simulink model "flightController"  (R2021a)
settings: Solver=ode3  StartTime=0  StopTime=10  FixedStep=Ts  RelTol=1e-3  EnableMultiTasking=on
undefined symbols (not defined in the file): Controller, ControlvsRed, D_ROLL, delays, DiscIntNeverNeededParam, g, I_ROLL, norm_act, Normalization, P_Pitch, P_ROLL, P_Roll, P_Yaw, P_z, PR_Start, save_time, sts_cnames, time_DisYaw, time_stepsX, time_stepsY, time_stepsZ, Ts, Vehicle, x0, x0_f
libraries: deeplib x5
(part 3 of 4)

== system flightController/Variant Subsystem/ANN/Subsystem2/Subsystem2 ==
  In1 : Inport
  Constant1 : Constant  Value=Ts
  Delay1 : Delay  DelayLength=1  InitialCondition=0
  Divide1 : Product  Inputs=*/
  Sum1 : Sum  Inputs=|+-
  Out1 : Outport
  wires:
  In1/1 -> Delay1/1, Sum1/1
  Constant1/1 -> Divide1/2
  Sum1/1 -> Divide1/1
  Delay1/1 -> Sum1/2
  Divide1/1 -> Out1/1

== system flightController/Variant Subsystem/ANN/Subsystem2/Subsystem3 ==
  In1 : Inport
  Bus Selector2 : BusSelector  OutputSignals=X,Y,Z,yaw,pitch,roll,dx,dy,dz,p,q,r
  Mux : Mux  Inputs=12
  Scope : Scope
  Out5 : Outport
  wires:
  In1/1 -> Bus Selector2/1
  Mux/1 -> Out5/1
  Bus Selector2/1 -> Mux/1  "<X>"
  Bus Selector2/2 -> Mux/2  "<Y>"
  Bus Selector2/3 -> Scope/1, Mux/3  "<Z>"
  Bus Selector2/4 -> Mux/4  "<yaw>"
  Bus Selector2/5 -> Mux/5  "<pitch>"
  Bus Selector2/6 -> Mux/6  "<roll>"
  Bus Selector2/7 -> Mux/7  "<dx>"
  Bus Selector2/8 -> Mux/8  "<dy>"
  Bus Selector2/9 -> Mux/9  "<dz>"
  Bus Selector2/10 -> Mux/10  "<p>"
  Bus Selector2/11 -> Mux/11  "<q>"
  Bus Selector2/12 -> Mux/12  "<r>"

== system flightController/Variant Subsystem/ANN_Feedback/Subsystem1/Subsystem ==
  note: Normalizacion de Sensores
  In1 : Inport
  Bus Selector2 : BusSelector  OutputSignals=ddx,ddy,ddz,p,q,r,altitude_sonar,prs
  Mux : Mux
  Subsystem1 : Subsystem  Commented=on
  Subsystem2 : Subsystem  Commented=on
  Subsystem3 : Subsystem  Commented=on
  Subsystem4 : Subsystem
  Subsystem5 : Subsystem
  Subsystem7 : Subsystem
  Subsystem8 : Subsystem  Commented=on
  Subsystem9 : Subsystem  Commented=on
  Ac_Dz : Outport
  wires:
  In1/1 -> Bus Selector2/1
  Bus Selector2/3 -> Subsystem7/1(<Ac_Dz>)  "<ddz>"
  Bus Selector2/4 -> Subsystem1/1(<Pressure Altitud>)  "<p>"
  Bus Selector2/7 -> Subsystem9/1(<Sonar Altitud>)  "<altitude_sonar>"
  Bus Selector2/8 -> Subsystem3/1(<Pressure Altitud>)  "<prs>"
  Bus Selector2/5 -> Subsystem8/1(<Pressure Altitud>)  "<q>"
  Bus Selector2/6 -> Subsystem2/1(<Pressure Altitud>)  "<r>"
  Mux/1 -> Ac_Dz/1
  Bus Selector2/2 -> Subsystem4/1(<Ac_Dz>)  "<ddy>"
  Bus Selector2/1 -> Subsystem5/1(<Ac_Dz>)  "<ddx>"
  Subsystem2/1(Pressure Altitud) -> Mux/4  "Gyro R"
  Subsystem7/1(Ac_Dz) -> Mux/3  "Ac_Dz"
  Subsystem4/1(Ac_Dz) -> Mux/2  "Ac_Dz"
  Subsystem5/1(Ac_Dz) -> Mux/1  "Ac_Dz"

== system flightController/Variant Subsystem/ANN_Feedback/Subsystem1/Subsystem10 ==
  note: Normalizacion de Sensores
  note: Normalizacion_Z
  note: Normalizacion de ref_Z
  note: Normalizacion_DZ
  note: Normalizacion_Acel_Z
  note: Normalizacion de ref_DZ
  In1 : Inport
  Bus Creator : BusCreator  Inputs=8
  Bus Selector : BusSelector  OutputSignals=Z,Dz,Z_r,Dz_r,Ac_Dz,Sonar Altitud,Pressure Altitud,Acceleracion Z
  Subsystem : Subsystem
  Subsystem2 : Subsystem
  Subsystem3 : Subsystem
  Subsystem4 : Subsystem
  Subsystem6 : Subsystem
  Subsystem7 : Subsystem
  Subsystem8 : Subsystem
  Subsystem9 : Subsystem
  Output : Outport
  wires:
  In1/1 -> Bus Selector/1
  Bus Selector/6 -> Subsystem9/1(<Sonar Altitud>)  "<Sonar Altitud>"
  Subsystem3/1(Z) -> Bus Creator/1
  Subsystem/1(Z_r) -> Bus Creator/3
  Subsystem9/1(Sonar Altitud) -> Bus Creator/6
  Subsystem6/1(Acceleracion Z) -> Bus Creator/8
  Bus Selector/1 -> Subsystem3/1(<Z>)  "<Z>"
  Subsystem7/1(Ac_Dz) -> Bus Creator/5
  Subsystem2/1(Dz_r) -> Bus Creator/4
  Bus Selector/3 -> Subsystem/1(<Z_r>)  "<Z_r>"
  Bus Selector/2 -> Subsystem4/1(<dz>)  "<Dz>"
  Subsystem4/1(Dz) -> Bus Creator/2
  Bus Selector/5 -> Subsystem7/1(<Ac_Dz>)  "<Ac_Dz>"
  Bus Creator/1 -> Output/1
  Subsystem8/1(Pressure Altitud) -> Bus Creator/7
  Bus Selector/4 -> Subsystem2/1(<Dz_r>)  "<Dz_r>"
  Bus Selector/7 -> Subsystem8/1(<Pressure Altitud>)  "<Pressure Altitud>"
  Bus Selector/8 -> Subsystem6/1(<Acel_z>)  "<Acceleracion Z>"

== system flightController/Variant Subsystem/ANN_Feedback/Subsystem1/Subsystem11 ==
  note: Normalizacion de ref_DZ
  note: Normalizacion_Z
  note: Normalizacion de ref_Z
  note: Normalizacion_Acel_Z
  note: Normalizacion de Sensores
  note: Normalizacion_DZ
  In1 : Inport
  Bus Creator : BusCreator  Inputs=8
  Bus Selector1 : BusSelector  OutputSignals=Z,Dz,Z_r,Dz_r,Ac_Dz,Sonar Altitud,Pressure Altitud,Acceleracion Z
  Subsystem : Subsystem
  Subsystem2 : Subsystem
  Subsystem3 : Subsystem
  Subsystem4 : Subsystem
  Subsystem6 : Subsystem
  Subsystem7 : Subsystem
  Subsystem8 : Subsystem
  Subsystem9 : Subsystem
  Output : Outport
  wires:
  Bus Selector1/4 -> Subsystem2/1(<Dz_r>)  "<Dz_r>"
  Bus Selector1/2 -> Subsystem4/1(<dz>)  "<Dz>"
  Bus Selector1/8 -> Subsystem6/1(<Acel_z>)  "<Acceleracion Z>"
  Bus Selector1/1 -> Subsystem3/1(<Z>)  "<Z>"
  In1/1 -> Bus Selector1/1
  Bus Selector1/7 -> Subsystem8/1(<Pressure Altitud>)  "<Pressure Altitud>"
  Subsystem8/1(Pressure Altitud) -> Bus Creator/7
  Subsystem4/1(Dz) -> Bus Creator/2
  Subsystem7/1(Ac_Dz) -> Bus Creator/5
  Bus Selector1/6 -> Subsystem9/1(<Sonar Altitud>)  "<Sonar Altitud>"
  Subsystem9/1(Sonar Altitud) -> Bus Creator/6
  Subsystem2/1(Dz_r) -> Bus Creator/4
  Subsystem6/1(Acceleracion Z) -> Bus Creator/8
  Bus Creator/1 -> Output/1
  Bus Selector1/5 -> Subsystem7/1(<Ac_Dz>)  "<Ac_Dz>"
  Bus Selector1/3 -> Subsystem/1(<Z_r>)  "<Z_r>"
  Subsystem3/1(Z) -> Bus Creator/1
  Subsystem/1(Z_r) -> Bus Creator/3

== system flightController/Variant Subsystem/ANN_Feedback/Subsystem1/Subsystem12 ==
  note: Normalizacion_DZ
  note: Normalizacion de Sensores
  note: Normalizacion_Acel_Z
  note: Normalizacion de ref_Z
  note: Normalizacion_Z
  note: Normalizacion de ref_DZ
  In1 : Inport
  Bus Creator : BusCreator  Inputs=8
  Bus Selector1 : BusSelector  OutputSignals=Z,Dz,Z_r,Dz_r,Ac_Dz,Sonar Altitud,Pressure Altitud,Acceleracion Z
  Subsystem : Subsystem
  Subsystem2 : Subsystem
  Subsystem3 : Subsystem
  Subsystem4 : Subsystem
  Subsystem6 : Subsystem
  Subsystem7 : Subsystem
  Subsystem8 : Subsystem
  Subsystem9 : Subsystem
  Output : Outport
  wires:
  Subsystem/1(Z_r) -> Bus Creator/3
  Subsystem3/1(Z) -> Bus Creator/1
  Bus Selector1/3 -> Subsystem/1(<Z_r>)  "<Z_r>"
  Bus Selector1/5 -> Subsystem7/1(<Ac_Dz>)  "<Ac_Dz>"
  Bus Creator/1 -> Output/1
  Subsystem6/1(Acceleracion Z) -> Bus Creator/8
  Subsystem2/1(Dz_r) -> Bus Creator/4
  Subsystem9/1(Sonar Altitud) -> Bus Creator/6
  Bus Selector1/6 -> Subsystem9/1(<Sonar Altitud>)  "<Sonar Altitud>"
  Subsystem7/1(Ac_Dz) -> Bus Creator/5
  Subsystem4/1(Dz) -> Bus Creator/2
  Subsystem8/1(Pressure Altitud) -> Bus Creator/7
  Bus Selector1/7 -> Subsystem8/1(<Pressure Altitud>)  "<Pressure Altitud>"
  In1/1 -> Bus Selector1/1
  Bus Selector1/1 -> Subsystem3/1(<Z>)  "<Z>"
  Bus Selector1/8 -> Subsystem6/1(<Acel_z>)  "<Acceleracion Z>"
  Bus Selector1/2 -> Subsystem4/1(<dz>)  "<Dz>"
  Bus Selector1/4 -> Subsystem2/1(<Dz_r>)  "<Dz_r>"

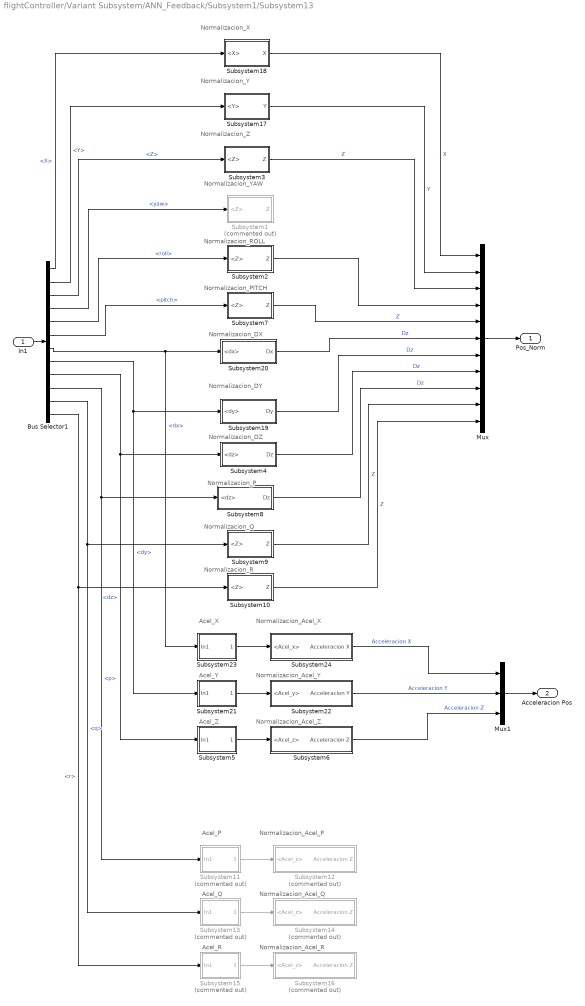
== system flightController/Variant Subsystem/ANN_Feedback/Subsystem1/Subsystem13 ==
  note: Acel_Z
  note: Normalizacion_DZ
  note: Normalizacion_Z
  note: Normalizacion_Acel_Z
  note: Normalizacion_YAW
  note: Normalizacion_ROLL
  note: Normalizacion_PITCH
  note: Normalizacion_P
  note: Normalizacion_Q
  note: Normalizacion_R
  note: Acel_P
  note: Normalizacion_Acel_P
  note: Acel_Q
  note: Normalizacion_Acel_Q
  note: Acel_R
  note: Normalizacion_Acel_R
  note: Normalizacion_Y
  note: Normalizacion_X
  note: Normalizacion_DY
  note: Normalizacion_DX
  note: Acel_Y
  note: Normalizacion_Acel_Y
  note: Acel_X
  note: Normalizacion_Acel_X
  In1 : Inport
  Bus Selector1 : BusSelector  OutputSignals=X,Y,Z,yaw,roll,pitch,dx,dy,dz,p,q,r
  Mux : Mux  Inputs=11
  Mux1 : Mux  Inputs=3
  Subsystem1 : Subsystem  Commented=on
  Subsystem10 : Subsystem
  Subsystem11 : Subsystem  Commented=on
  Subsystem12 : Subsystem  Commented=on
  Subsystem13 : Subsystem  Commented=on
  Subsystem14 : Subsystem  Commented=on
  Subsystem15 : Subsystem  Commented=on
  Subsystem16 : Subsystem  Commented=on
  Subsystem17 : Subsystem
  Subsystem18 : Subsystem
  Subsystem19 : Subsystem
  Subsystem2 : Subsystem
  Subsystem20 : Subsystem
  Subsystem21 : Subsystem
  Subsystem22 : Subsystem
  Subsystem23 : Subsystem
  Subsystem24 : Subsystem
  Subsystem3 : Subsystem
  Subsystem4 : Subsystem
  Subsystem5 : Subsystem
  Subsystem6 : Subsystem
  Subsystem7 : Subsystem
  Subsystem8 : Subsystem
  Subsystem9 : Subsystem
  Pos_Norm : Outport
  Acceleracion Pos : Outport  Port=2
  wires:
  Bus Selector1/3 -> Subsystem3/1(<Z>)  "<Z>"
  Bus Selector1/9 -> Subsystem5/1(In1), Subsystem4/1(<dz>)  "<dz>"
  Subsystem5/1(<Acel_Z>) -> Subsystem6/1(<Acel_z>)
  In1/1 -> Bus Selector1/1
  Bus Selector1/4 -> Subsystem1/1(<Z>)  "<yaw>"
  Bus Selector1/10 -> Subsystem8/1(<dz>), Subsystem11/1(In1)  "<p>"
  Bus Selector1/11 -> Subsystem9/1(<Z>), Subsystem13/1(In1)  "<q>"
  Bus Selector1/12 -> Subsystem10/1(<Z>), Subsystem15/1(In1)  "<r>"
  Mux/1 -> Pos_Norm/1
  Mux1/1 -> Acceleracion Pos/1
  Subsystem11/1(<Acel_Z>) -> Subsystem12/1(<Acel_z>)
  Subsystem13/1(<Acel_Z>) -> Subsystem14/1(<Acel_z>)
  Subsystem15/1(<Acel_Z>) -> Subsystem16/1(<Acel_z>)
  Bus Selector1/5 -> Subsystem2/1(<Z>)  "<roll>"
  Bus Selector1/6 -> Subsystem7/1(<Z>)  "<pitch>"
  Bus Selector1/2 -> Subsystem17/1(<Y>)  "<Y>"
  Bus Selector1/1 -> Subsystem18/1(<X>)  "<X>"
  Bus Selector1/7 -> Subsystem23/1(In1), Subsystem20/1(<dx>)  "<dx>"
  Bus Selector1/8 -> Subsystem21/1(In1), Subsystem19/1(<dy>)  "<dy>"
  Subsystem18/1(X) -> Mux/1  "X"
  Subsystem17/1(Y) -> Mux/2  "Y"
  Subsystem3/1(Z) -> Mux/3  "Z"
  Subsystem2/1(Z) -> Mux/4
  Subsystem7/1(Z) -> Mux/5  "Z"
  Subsystem20/1(Dx) -> Mux/6  "Dz"
  Subsystem19/1(Dy) -> Mux/7  "Dz"
  Subsystem4/1(Dz) -> Mux/8  "Dz"
  Subsystem8/1(Dz) -> Mux/9  "Dz"
  Subsystem9/1(Z) -> Mux/10  "Z"
  Subsystem10/1(Z) -> Mux/11  "Z"
  Subsystem21/1(<Acel_Y>) -> Subsystem22/1(<Acel_y>)
  Subsystem23/1(<Acel_X>) -> Subsystem24/1(<Acel_x>)
  Subsystem22/1(Acceleracion Y) -> Mux1/2  "Acceleracion Y"
  Subsystem24/1(Acceleracion X) -> Mux1/1  "Acceleracion X"
  Subsystem6/1(Acceleracion Z) -> Mux1/3  "Acceleracion Z"

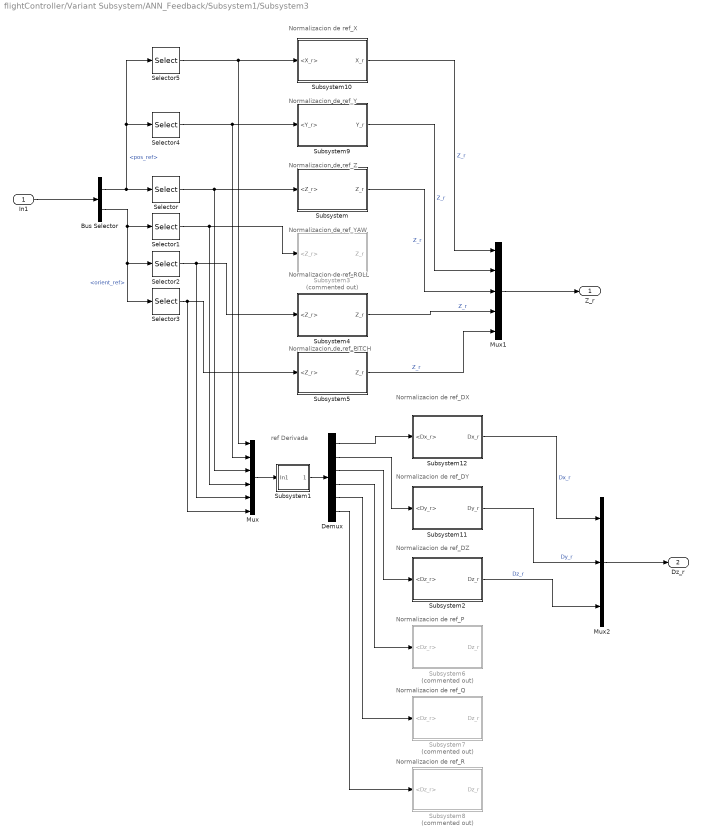
== system flightController/Variant Subsystem/ANN_Feedback/Subsystem1/Subsystem3 ==
  note: Normalizacion de ref_Z
  note: ref
      | Derivada
  note: Normalizacion de ref_DZ
  note: Normalizacion de ref_YAW
  note: Normalizacion de ref_ROLL
  note: Normalizacion de ref_PITCH
  note: Normalizacion de ref_P
  note: Normalizacion de ref_Q
  note: Normalizacion de ref_R
  note: Normalizacion de ref_Y
  note: Normalizacion de ref_X
  note: Normalizacion de ref_DY
  note: Normalizacion de ref_DX
  In1 : Inport
  Bus Selector : BusSelector  OutputSignals=pos_ref,orient_ref
  Demux : Demux  Outputs=6
  Mux : Mux  Inputs=6
  Mux1 : Mux  Inputs=5
  Mux2 : Mux  Inputs=3
  Selector : Selector  InputPortWidth=3  IndexOptions=Index vector (dialog)  Indices=[3]  OutputSizes=1
  Selector1 : Selector  InputPortWidth=3  IndexOptions=Index vector (dialog)  Indices=[1]  OutputSizes=1
  Selector2 : Selector  InputPortWidth=3  IndexOptions=Index vector (dialog)  Indices=[3]  OutputSizes=1
  Selector3 : Selector  InputPortWidth=3  IndexOptions=Index vector (dialog)  Indices=[2]  OutputSizes=1
  Selector4 : Selector  InputPortWidth=3  IndexOptions=Index vector (dialog)  Indices=[2]  OutputSizes=1
  Selector5 : Selector  InputPortWidth=3  IndexOptions=Index vector (dialog)  Indices=[1]  OutputSizes=1
  Subsystem : Subsystem
  Subsystem1 : Subsystem
  Subsystem10 : Subsystem
  Subsystem11 : Subsystem
  Subsystem12 : Subsystem
  Subsystem2 : Subsystem
  Subsystem3 : Subsystem  Commented=on
  Subsystem4 : Subsystem
  Subsystem5 : Subsystem
  Subsystem6 : Subsystem  Commented=on
  Subsystem7 : Subsystem  Commented=on
  Subsystem8 : Subsystem  Commented=on
  Subsystem9 : Subsystem
  Z_r : Outport
  Dz_r : Outport  Port=2
  wires:
  Bus Selector/1 -> Selector5/1, Selector4/1, Selector/1  "<pos_ref>"
  Selector/1 -> Subsystem/1(<Z_r>), Mux/3
  In1/1 -> Bus Selector/1
  Bus Selector/2 -> Selector2/1, Selector3/1, Selector1/1  "<orient_ref>"
  Selector1/1 -> Mux/4, Subsystem3/1(<Z_r>)
  Selector2/1 -> Mux/5, Subsystem4/1(<Z_r>)
  Selector3/1 -> Mux/6, Subsystem5/1(<Z_r>)
  Mux/1 -> Subsystem1/1(In1)
  Subsystem1/1(Out1) -> Demux/1
  Mux1/1 -> Z_r/1
  Mux2/1 -> Dz_r/1
  Selector4/1 -> Mux/2, Subsystem9/1(<Y_r>)
  Selector5/1 -> Mux/1, Subsystem10/1(<X_r>)
  Subsystem10/1(X_r) -> Mux1/1  "Z_r"
  Subsystem9/1(Y_r) -> Mux1/2  "Z_r"
  Subsystem/1(Z_r) -> Mux1/3  "Z_r"
  Subsystem4/1(Z_r) -> Mux1/4  "Z_r"
  Subsystem5/1(Z_r) -> Mux1/5  "Z_r"
  Demux/1 -> Subsystem12/1(<Dx_r>)
  Demux/2 -> Subsystem11/1(<Dy_r>)
  Demux/3 -> Subsystem2/1(<Dz_r>)
  Subsystem12/1(Dx_r) -> Mux2/1  "Dx_r"
  Subsystem11/1(Dy_r) -> Mux2/2  "Dy_r"
  Subsystem2/1(Dz_r) -> Mux2/3  "Dz_r"
  Demux/4 -> Subsystem6/1(<Dz_r>)
  Demux/5 -> Subsystem7/1(<Dz_r>)
  Demux/6 -> Subsystem8/1(<Dz_r>)

== system flightController/Variant Subsystem/ANN_Feedback/Subsystem2/Subsystem ==
  In1 : Inport
  Bus Selector2 : BusSelector  OutputSignals=ddx,ddy,ddz,p,q,r,altitude_sonar,prs,vbat_V,vbat_percentage
  Cast To Single : DataTypeConversion  OutDataTypeStr=single
  Mux : Mux  Inputs=10
  Scope : Scope
  Out5 : Outport
  wires:
  In1/1 -> Bus Selector2/1
  Bus Selector2/1 -> Mux/1  "<ddx>"
  Bus Selector2/2 -> Mux/2  "<ddy>"
  Bus Selector2/3 -> Mux/3  "<ddz>"
  Bus Selector2/4 -> Mux/4  "<p>"
  Bus Selector2/5 -> Mux/5  "<q>"
  Bus Selector2/6 -> Mux/6  "<r>"
  Bus Selector2/7 -> Mux/7  "<altitude_sonar>"
  Bus Selector2/8 -> Mux/8  "<prs>"
  Bus Selector2/9 -> Mux/9  "<vbat_V>"
  Mux/1 -> Scope/1, Out5/1
  Bus Selector2/10 -> Cast To Single/1  "<vbat_percentage>"
  Cast To Single/1 -> Mux/10

== system flightController/Variant Subsystem/ANN_Feedback/Subsystem2/Subsystem1 ==
  In1 : Inport
  Constant1 : Constant  Value=Ts
  Delay1 : Delay  DelayLength=1  InitialCondition=0
  Divide1 : Product  Inputs=*/
  Sum1 : Sum  Inputs=|+-
  Out1 : Outport
  wires:
  In1/1 -> Delay1/1, Sum1/1
  Constant1/1 -> Divide1/2
  Sum1/1 -> Divide1/1
  Delay1/1 -> Sum1/2
  Divide1/1 -> Out1/1

== system flightController/Variant Subsystem/ANN_Feedback/Subsystem2/Subsystem2 ==
  In1 : Inport
  Constant1 : Constant  Value=Ts
  Delay1 : Delay  DelayLength=1  InitialCondition=0
  Divide1 : Product  Inputs=*/
  Sum1 : Sum  Inputs=|+-
  Out1 : Outport
  wires:
  In1/1 -> Delay1/1, Sum1/1
  Constant1/1 -> Divide1/2
  Sum1/1 -> Divide1/1
  Delay1/1 -> Sum1/2
  Divide1/1 -> Out1/1

== system flightController/Variant Subsystem/ANN_Feedback/Subsystem2/Subsystem3 ==
  In1 : Inport
  Bus Selector2 : BusSelector  OutputSignals=X,Y,Z,yaw,pitch,roll,dx,dy,dz,p,q,r
  Mux : Mux  Inputs=12
  Scope : Scope
  Out5 : Outport
  wires:
  In1/1 -> Bus Selector2/1
  Mux/1 -> Out5/1
  Bus Selector2/1 -> Mux/1  "<X>"
  Bus Selector2/2 -> Mux/2  "<Y>"
  Bus Selector2/3 -> Scope/1, Mux/3  "<Z>"
  Bus Selector2/4 -> Mux/4  "<yaw>"
  Bus Selector2/5 -> Mux/5  "<pitch>"
  Bus Selector2/6 -> Mux/6  "<roll>"
  Bus Selector2/7 -> Mux/7  "<dx>"
  Bus Selector2/8 -> Mux/8  "<dy>"
  Bus Selector2/9 -> Mux/9  "<dz>"
  Bus Selector2/10 -> Mux/10  "<p>"
  Bus Selector2/11 -> Mux/11  "<q>"
  Bus Selector2/12 -> Mux/12  "<r>"

== system flightController/Variant Subsystem/LSTM/Subsystem2/Subsystem ==
  In1 : Inport
  Bus Selector2 : BusSelector  OutputSignals=ddx,ddy,ddz,p,q,r,altitude_sonar,prs,vbat_V,vbat_percentage
  Cast To Single : DataTypeConversion  OutDataTypeStr=single
  Mux : Mux  Inputs=10
  Scope : Scope
  Out5 : Outport
  wires:
  In1/1 -> Bus Selector2/1
  Bus Selector2/1 -> Mux/1  "<ddx>"
  Bus Selector2/2 -> Mux/2  "<ddy>"
  Bus Selector2/3 -> Mux/3  "<ddz>"
  Bus Selector2/4 -> Mux/4  "<p>"
  Bus Selector2/5 -> Mux/5  "<q>"
  Bus Selector2/6 -> Mux/6  "<r>"
  Bus Selector2/7 -> Mux/7  "<altitude_sonar>"
  Bus Selector2/8 -> Mux/8  "<prs>"
  Bus Selector2/9 -> Mux/9  "<vbat_V>"
  Mux/1 -> Scope/1, Out5/1
  Bus Selector2/10 -> Cast To Single/1  "<vbat_percentage>"
  Cast To Single/1 -> Mux/10

== system flightController/Variant Subsystem/LSTM/Subsystem2/Subsystem1 ==
  In1 : Inport
  Constant1 : Constant  Value=Ts
  Delay1 : Delay  DelayLength=1  InitialCondition=0
  Divide1 : Product  Inputs=*/
  Sum1 : Sum  Inputs=|+-
  Out1 : Outport
  wires:
  In1/1 -> Delay1/1, Sum1/1
  Constant1/1 -> Divide1/2
  Sum1/1 -> Divide1/1
  Delay1/1 -> Sum1/2
  Divide1/1 -> Out1/1

== system flightController/Variant Subsystem/LSTM/Subsystem2/Subsystem2 ==
  In1 : Inport
  Constant1 : Constant  Value=Ts
  Delay1 : Delay  DelayLength=1  InitialCondition=0
  Divide1 : Product  Inputs=*/
  Sum1 : Sum  Inputs=|+-
  Out1 : Outport
  wires:
  In1/1 -> Delay1/1, Sum1/1
  Constant1/1 -> Divide1/2
  Sum1/1 -> Divide1/1
  Delay1/1 -> Sum1/2
  Divide1/1 -> Out1/1

== system flightController/Variant Subsystem/LSTM/Subsystem2/Subsystem3 ==
  In1 : Inport
  Bus Selector2 : BusSelector  OutputSignals=X,Y,Z,yaw,pitch,roll,dx,dy,dz,p,q,r
  Mux : Mux  Inputs=12
  Scope : Scope
  Out5 : Outport
  wires:
  In1/1 -> Bus Selector2/1
  Mux/1 -> Out5/1
  Bus Selector2/1 -> Mux/1  "<X>"
  Bus Selector2/2 -> Mux/2  "<Y>"
  Bus Selector2/3 -> Scope/1, Mux/3  "<Z>"
  Bus Selector2/4 -> Mux/4  "<yaw>"
  Bus Selector2/7 -> Mux/7  "<dx>"
  Bus Selector2/8 -> Mux/8  "<dy>"
  Bus Selector2/9 -> Mux/9  "<dz>"
  Bus Selector2/10 -> Mux/10  "<p>"
  Bus Selector2/11 -> Mux/11  "<q>"
  Bus Selector2/12 -> Mux/12  "<r>"
  Bus Selector2/6 -> Mux/5  "<roll>"
  Bus Selector2/5 -> Mux/6  "<pitch>"

== system flightController/Variant Subsystem/LSTM/Subsystem3/Subsystem ==
  In1 : Inport
  Bus Selector2 : BusSelector  OutputSignals=ddx,ddy,ddz,p,q,r,altitude_sonar,prs,vbat_V,vbat_percentage
  Cast To Single : DataTypeConversion  OutDataTypeStr=single
  Mux : Mux  Inputs=10
  Out5 : Outport
  wires:
  In1/1 -> Bus Selector2/1
  Bus Selector2/1 -> Mux/1  "<ddx>"
  Bus Selector2/2 -> Mux/2  "<ddy>"
  Bus Selector2/3 -> Mux/3  "<ddz>"
  Bus Selector2/4 -> Mux/4  "<p>"
  Bus Selector2/5 -> Mux/5  "<q>"
  Bus Selector2/6 -> Mux/6  "<r>"
  Bus Selector2/7 -> Mux/7  "<altitude_sonar>"
  Bus Selector2/8 -> Mux/8  "<prs>"
  Bus Selector2/9 -> Mux/9  "<vbat_V>"
  Mux/1 -> Out5/1
  Bus Selector2/10 -> Cast To Single/1  "<vbat_percentage>"
  Cast To Single/1 -> Mux/10

== system flightController/Variant Subsystem/LSTM/Subsystem3/Subsystem1 ==
  In1 : Inport
  Constant1 : Constant  Value=Ts
  Delay1 : Delay  DelayLength=1  InitialCondition=0
  Divide1 : Product  Inputs=*/
  Sum1 : Sum  Inputs=|+-
  Out1 : Outport
  wires:
  In1/1 -> Delay1/1, Sum1/1
  Constant1/1 -> Divide1/2
  Sum1/1 -> Divide1/1
  Delay1/1 -> Sum1/2
  Divide1/1 -> Out1/1

== system flightController/Variant Subsystem/LSTM/Subsystem3/Subsystem2 ==
  In1 : Inport
  Constant1 : Constant  Value=Ts
  Delay1 : Delay  DelayLength=1  InitialCondition=0
  Divide1 : Product  Inputs=*/
  Sum1 : Sum  Inputs=|+-
  Out1 : Outport
  wires:
  In1/1 -> Delay1/1, Sum1/1
  Constant1/1 -> Divide1/2
  Sum1/1 -> Divide1/1
  Delay1/1 -> Sum1/2
  Divide1/1 -> Out1/1

== system flightController/Variant Subsystem/LSTM/Subsystem3/Subsystem3 ==
  In1 : Inport
  Bus Selector2 : BusSelector  OutputSignals=X,Y,Z,yaw,pitch,roll,dx,dy,dz,p,q,r
  Mux : Mux  Inputs=12
  Scope : Scope
  Out5 : Outport
  wires:
  In1/1 -> Bus Selector2/1
  Mux/1 -> Out5/1
  Bus Selector2/1 -> Mux/1  "<X>"
  Bus Selector2/2 -> Mux/2  "<Y>"
  Bus Selector2/3 -> Scope/1, Mux/3  "<Z>"
  Bus Selector2/4 -> Mux/4  "<yaw>"
  Bus Selector2/5 -> Mux/5  "<pitch>"
  Bus Selector2/6 -> Mux/6  "<roll>"
  Bus Selector2/7 -> Mux/7  "<dx>"
  Bus Selector2/8 -> Mux/8  "<dy>"
  Bus Selector2/9 -> Mux/9  "<dz>"
  Bus Selector2/10 -> Mux/10  "<p>"
  Bus Selector2/11 -> Mux/11  "<q>"
  Bus Selector2/12 -> Mux/12  "<r>"

== system flightController/Variant Subsystem/ANN/Subsystem/Subsystem/Subsystem1 ==
  <Pressure Altitud> : Inport
  Constant : Constant  Value=Normalization(13,2)
  Gain : Gain  Gain=1/(Normalization(13,1)-Normalization(13,2))
  Sum : Sum  Inputs=|+-
  Pressure Altitud : Outport
  wires:
  <Pressure Altitud>/1 -> Sum/1
  Sum/1 -> Gain/1
  Constant/1 -> Sum/2
  Gain/1 -> Pressure Altitud/1

== system flightController/Variant Subsystem/ANN/Subsystem/Subsystem/Subsystem2 ==
  <Pressure Altitud> : Inport
  Constant : Constant  Value=Normalization(15,2)
  Gain : Gain  Gain=1/(Normalization(15,1)-Normalization(15,2))
  Sum : Sum  Inputs=|+-
  Pressure Altitud : Outport
  wires:
  <Pressure Altitud>/1 -> Sum/1
  Sum/1 -> Gain/1
  Constant/1 -> Sum/2
  Gain/1 -> Pressure Altitud/1

== system flightController/Variant Subsystem/ANN/Subsystem/Subsystem/Subsystem3 ==
  <Pressure Altitud> : Inport
  Constant : Constant  Value=Normalization(17,2)
  Gain : Gain  Gain=1/(Normalization(17,1)-Normalization(17,2))
  Sum : Sum  Inputs=|+-
  Pressure Altitud : Outport
  wires:
  <Pressure Altitud>/1 -> Sum/1
  Sum/1 -> Gain/1
  Constant/1 -> Sum/2
  Gain/1 -> Pressure Altitud/1

== system flightController/Variant Subsystem/ANN/Subsystem/Subsystem/Subsystem7 ==
  <Ac_Dz> : Inport
  Constant : Constant  Value=Normalization(12,2)
  Gain : Gain  Gain=1/(Normalization(12,1)-Normalization(12,2))
  Sum : Sum  Inputs=|+-
  Ac_Dz : Outport
  wires:
  <Ac_Dz>/1 -> Sum/1
  Sum/1 -> Gain/1
  Constant/1 -> Sum/2
  Gain/1 -> Ac_Dz/1

== system flightController/Variant Subsystem/ANN/Subsystem/Subsystem/Subsystem8 ==
  <Pressure Altitud> : Inport
  Constant : Constant  Value=Normalization(14,2)
  Gain : Gain  Gain=1/(Normalization(14,1)-Normalization(14,2))
  Sum : Sum  Inputs=|+-
  Pressure Altitud : Outport
  wires:
  <Pressure Altitud>/1 -> Sum/1
  Sum/1 -> Gain/1
  Constant/1 -> Sum/2
  Gain/1 -> Pressure Altitud/1

== system flightController/Variant Subsystem/ANN/Subsystem/Subsystem/Subsystem9 ==
  <Sonar Altitud> : Inport
  Constant : Constant  Value=Normalization(16,2)
  Gain : Gain  Gain=1/(Normalization(16,1)-Normalization(16,2))
  Scope : Scope
  Sum : Sum  Inputs=|+-
  Sonar Altitud : Outport
  wires:
  <Sonar Altitud>/1 -> Scope/1, Sum/1
  Sum/1 -> Gain/1
  Constant/1 -> Sum/2
  Gain/1 -> Sonar Altitud/1

== system flightController/Variant Subsystem/ANN/Subsystem/Subsystem10/Subsystem ==
  <Z_r> : Inport
  Constant : Constant  Value=Normalization(10,2)
  Gain : Gain  Gain=1/(Normalization(10,1)-Normalization(10,2))
  Sum : Sum  Inputs=|+-
  Z_r : Outport
  wires:
  <Z_r>/1 -> Sum/1
  Sum/1 -> Gain/1
  Constant/1 -> Sum/2
  Gain/1 -> Z_r/1

== system flightController/Variant Subsystem/ANN/Subsystem/Subsystem10/Subsystem2 ==
  <Dz_r> : Inport
  Constant : Constant  Value=Normalization(14,2)
  Gain : Gain  Gain=1/(Normalization(14,1)-Normalization(14,2))
  Sum : Sum  Inputs=|+-
  Dz_r : Outport
  wires:
  <Dz_r>/1 -> Sum/1
  Sum/1 -> Gain/1
  Constant/1 -> Sum/2
  Gain/1 -> Dz_r/1

== system flightController/Variant Subsystem/ANN/Subsystem/Subsystem10/Subsystem3 ==
  <Z> : Inport
  Constant : Constant  Value=Normalization(2,2)
  Gain : Gain  Gain=1/(Normalization(2,1)-Normalization(2,2))
  Sum : Sum  Inputs=|+-
  Z : Outport
  wires:
  Constant/1 -> Sum/2
  Sum/1 -> Gain/1
  Gain/1 -> Z/1
  <Z>/1 -> Sum/1

== system flightController/Variant Subsystem/ANN/Subsystem/Subsystem10/Subsystem4 ==
  <dz> : Inport
  Constant : Constant  Value=Normalization(5,2)
  Gain : Gain  Gain=1/(Normalization(5,1)-Normalization(5,2))
  Sum : Sum  Inputs=|+-
  Dz : Outport
  wires:
  Gain/1 -> Dz/1
  Constant/1 -> Sum/2
  <dz>/1 -> Sum/1
  Sum/1 -> Gain/1

== system flightController/Variant Subsystem/ANN/Subsystem/Subsystem10/Subsystem6 ==
  <Acel_z> : Inport
  Constant : Constant  Value=Normalization(30,2)
  Gain : Gain  Gain=1/(Normalization(30,1)-Normalization(30,2))
  Sum : Sum  Inputs=|+-
  Acceleracion Z : Outport
  wires:
  Gain/1 -> Acceleracion Z/1
  Constant/1 -> Sum/2
  <Acel_z>/1 -> Sum/1
  Sum/1 -> Gain/1

== system flightController/Variant Subsystem/ANN/Subsystem/Subsystem10/Subsystem7 ==
  <Ac_Dz> : Inport
  Constant : Constant  Value=Normalization(18,2)
  Gain : Gain  Gain=1/(Normalization(18,1)-Normalization(18,2))
  Sum : Sum  Inputs=|+-
  Ac_Dz : Outport
  wires:
  <Ac_Dz>/1 -> Sum/1
  Sum/1 -> Gain/1
  Constant/1 -> Sum/2
  Gain/1 -> Ac_Dz/1

== system flightController/Variant Subsystem/ANN/Subsystem/Subsystem10/Subsystem8 ==
  <Pressure Altitud> : Inport
  Constant : Constant  Value=Normalization(26,2)
  Gain : Gain  Gain=1/(Normalization(26,1)-Normalization(26,2))
  Sum : Sum  Inputs=|+-
  Pressure Altitud : Outport
  wires:
  <Pressure Altitud>/1 -> Sum/1
  Sum/1 -> Gain/1
  Constant/1 -> Sum/2
  Gain/1 -> Pressure Altitud/1

== system flightController/Variant Subsystem/ANN/Subsystem/Subsystem10/Subsystem9 ==
  <Sonar Altitud> : Inport
  Constant : Constant  Value=Normalization(22,2)
  Gain : Gain  Gain=1/(Normalization(22,1)-Normalization(22,2))
  Sum : Sum  Inputs=|+-
  Sonar Altitud : Outport
  wires:
  <Sonar Altitud>/1 -> Sum/1
  Sum/1 -> Gain/1
  Constant/1 -> Sum/2
  Gain/1 -> Sonar Altitud/1

== system flightController/Variant Subsystem/ANN/Subsystem/Subsystem11/Subsystem ==
  <Z_r> : Inport
  Constant : Constant  Value=Normalization(10,2)
  Gain : Gain  Gain=1/(Normalization(10,1)-Normalization(10,2))
  Sum : Sum  Inputs=|+-
  Z_r : Outport
  wires:
  <Z_r>/1 -> Sum/1
  Sum/1 -> Gain/1
  Constant/1 -> Sum/2
  Gain/1 -> Z_r/1

== system flightController/Variant Subsystem/ANN/Subsystem/Subsystem11/Subsystem2 ==
  <Dz_r> : Inport
  Constant : Constant  Value=Normalization(14,2)
  Gain : Gain  Gain=1/(Normalization(14,1)-Normalization(14,2))
  Sum : Sum  Inputs=|+-
  Dz_r : Outport
  wires:
  <Dz_r>/1 -> Sum/1
  Sum/1 -> Gain/1
  Constant/1 -> Sum/2
  Gain/1 -> Dz_r/1

== system flightController/Variant Subsystem/ANN/Subsystem/Subsystem11/Subsystem3 ==
  <Z> : Inport
  Constant : Constant  Value=Normalization(3,2)
  Gain : Gain  Gain=1/(Normalization(3,1)-Normalization(3,2))
  Sum : Sum  Inputs=|+-
  Z : Outport
  wires:
  Constant/1 -> Sum/2
  Sum/1 -> Gain/1
  Gain/1 -> Z/1
  <Z>/1 -> Sum/1

== system flightController/Variant Subsystem/ANN/Subsystem/Subsystem11/Subsystem4 ==
  <dz> : Inport
  Constant : Constant  Value=Normalization(6,2)
  Gain : Gain  Gain=1/(Normalization(6,1)-Normalization(6,2))
  Sum : Sum  Inputs=|+-
  Dz : Outport
  wires:
  Gain/1 -> Dz/1
  Constant/1 -> Sum/2
  <dz>/1 -> Sum/1
  Sum/1 -> Gain/1

== system flightController/Variant Subsystem/ANN/Subsystem/Subsystem11/Subsystem6 ==
  <Acel_z> : Inport
  Constant : Constant  Value=Normalization(30,2)
  Gain : Gain  Gain=1/(Normalization(30,1)-Normalization(30,2))
  Sum : Sum  Inputs=|+-
  Acceleracion Z : Outport
  wires:
  Gain/1 -> Acceleracion Z/1
  Constant/1 -> Sum/2
  <Acel_z>/1 -> Sum/1
  Sum/1 -> Gain/1

== system flightController/Variant Subsystem/ANN/Subsystem/Subsystem11/Subsystem7 ==
  <Ac_Dz> : Inport
  Constant : Constant  Value=Normalization(18,2)
  Gain : Gain  Gain=1/(Normalization(18,1)-Normalization(18,2))
  Sum : Sum  Inputs=|+-
  Ac_Dz : Outport
  wires:
  <Ac_Dz>/1 -> Sum/1
  Sum/1 -> Gain/1
  Constant/1 -> Sum/2
  Gain/1 -> Ac_Dz/1

== system flightController/Variant Subsystem/ANN/Subsystem/Subsystem11/Subsystem8 ==
  <Pressure Altitud> : Inport
  Constant : Constant  Value=Normalization(26,2)
  Gain : Gain  Gain=1/(Normalization(26,1)-Normalization(26,2))
  Sum : Sum  Inputs=|+-
  Pressure Altitud : Outport
  wires:
  <Pressure Altitud>/1 -> Sum/1
  Sum/1 -> Gain/1
  Constant/1 -> Sum/2
  Gain/1 -> Pressure Altitud/1

== system flightController/Variant Subsystem/ANN/Subsystem/Subsystem11/Subsystem9 ==
  <Sonar Altitud> : Inport
  Constant : Constant  Value=Normalization(22,2)
  Gain : Gain  Gain=1/(Normalization(22,1)-Normalization(22,2))
  Sum : Sum  Inputs=|+-
  Sonar Altitud : Outport
  wires:
  <Sonar Altitud>/1 -> Sum/1
  Sum/1 -> Gain/1
  Constant/1 -> Sum/2
  Gain/1 -> Sonar Altitud/1

== system flightController/Variant Subsystem/ANN/Subsystem/Subsystem12/Subsystem ==
  <Z_r> : Inport
  Constant : Constant  Value=Normalization(10,2)
  Gain : Gain  Gain=1/(Normalization(10,1)-Normalization(10,2))
  Sum : Sum  Inputs=|+-
  Z_r : Outport
  wires:
  Gain/1 -> Z_r/1
  Constant/1 -> Sum/2
  Sum/1 -> Gain/1
  <Z_r>/1 -> Sum/1

== system flightController/Variant Subsystem/ANN/Subsystem/Subsystem12/Subsystem2 ==
  <Dz_r> : Inport
  Constant : Constant  Value=Normalization(14,2)
  Gain : Gain  Gain=1/(Normalization(14,1)-Normalization(14,2))
  Sum : Sum  Inputs=|+-
  Dz_r : Outport
  wires:
  Gain/1 -> Dz_r/1
  Constant/1 -> Sum/2
  Sum/1 -> Gain/1
  <Dz_r>/1 -> Sum/1

== system flightController/Variant Subsystem/ANN/Subsystem/Subsystem12/Subsystem3 ==
  <Z> : Inport
  Constant : Constant  Value=Normalization(3,2)
  Gain : Gain  Gain=1/(Normalization(3,1)-Normalization(3,2))
  Sum : Sum  Inputs=|+-
  Z : Outport
  wires:
  <Z>/1 -> Sum/1
  Gain/1 -> Z/1
  Sum/1 -> Gain/1
  Constant/1 -> Sum/2

== system flightController/Variant Subsystem/ANN/Subsystem/Subsystem12/Subsystem4 ==
  <dz> : Inport
  Constant : Constant  Value=Normalization(6,2)
  Gain : Gain  Gain=1/(Normalization(6,1)-Normalization(6,2))
  Sum : Sum  Inputs=|+-
  Dz : Outport
  wires:
  Sum/1 -> Gain/1
  <dz>/1 -> Sum/1
  Constant/1 -> Sum/2
  Gain/1 -> Dz/1

== system flightController/Variant Subsystem/ANN/Subsystem/Subsystem12/Subsystem6 ==
  <Acel_z> : Inport
  Constant : Constant  Value=Normalization(30,2)
  Gain : Gain  Gain=1/(Normalization(30,1)-Normalization(30,2))
  Sum : Sum  Inputs=|+-
  Acceleracion Z : Outport
  wires:
  Sum/1 -> Gain/1
  <Acel_z>/1 -> Sum/1
  Constant/1 -> Sum/2
  Gain/1 -> Acceleracion Z/1

== system flightController/Variant Subsystem/ANN/Subsystem/Subsystem12/Subsystem7 ==
  <Ac_Dz> : Inport
  Constant : Constant  Value=Normalization(18,2)
  Gain : Gain  Gain=1/(Normalization(18,1)-Normalization(18,2))
  Sum : Sum  Inputs=|+-
  Ac_Dz : Outport
  wires:
  Gain/1 -> Ac_Dz/1
  Constant/1 -> Sum/2
  Sum/1 -> Gain/1
  <Ac_Dz>/1 -> Sum/1

== system flightController/Variant Subsystem/ANN/Subsystem/Subsystem12/Subsystem8 ==
  <Pressure Altitud> : Inport
  Constant : Constant  Value=Normalization(26,2)
  Gain : Gain  Gain=1/(Normalization(26,1)-Normalization(26,2))
  Sum : Sum  Inputs=|+-
  Pressure Altitud : Outport
  wires:
  Gain/1 -> Pressure Altitud/1
  Constant/1 -> Sum/2
  Sum/1 -> Gain/1
  <Pressure Altitud>/1 -> Sum/1

== system flightController/Variant Subsystem/ANN/Subsystem/Subsystem12/Subsystem9 ==
  <Sonar Altitud> : Inport
  Constant : Constant  Value=Normalization(22,2)
  Gain : Gain  Gain=1/(Normalization(22,1)-Normalization(22,2))
  Sum : Sum  Inputs=|+-
  Sonar Altitud : Outport
  wires:
  Gain/1 -> Sonar Altitud/1
  Constant/1 -> Sum/2
  Sum/1 -> Gain/1
  <Sonar Altitud>/1 -> Sum/1

== system flightController/Variant Subsystem/ANN/Subsystem/Subsystem13/Subsystem1 ==
  <Z> : Inport
  Constant : Constant  Value=Normalization(2,2)
  Gain : Gain  Gain=1/(Normalization(2,1)-Normalization(2,2))
  Sum : Sum  Inputs=|+-
  Z : Outport
  wires:
  Constant/1 -> Sum/2
  Sum/1 -> Gain/1
  Gain/1 -> Z/1
  <Z>/1 -> Sum/1

== system flightController/Variant Subsystem/ANN/Subsystem/Subsystem13/Subsystem10 ==
  <Z> : Inport
  Constant : Constant  Value=Normalization(7,2)
  Gain : Gain  Gain=1/(Normalization(7,1)-Normalization(7,2))
  Sum : Sum  Inputs=|+-
  Z : Outport
  wires:
  Constant/1 -> Sum/2
  Sum/1 -> Gain/1
  Gain/1 -> Z/1
  <Z>/1 -> Sum/1

== system flightController/Variant Subsystem/ANN/Subsystem/Subsystem13/Subsystem11 ==
  In1 : Inport
  Constant1 : Constant  Value=Ts
  Delay1 : Delay  DelayLength=1  InitialCondition=0
  Divide1 : Product  Inputs=*/
  Sum1 : Sum  Inputs=|+-
  <Acel_Z> : Outport
  wires:
  Divide1/1 -> <Acel_Z>/1
  Delay1/1 -> Sum1/2
  Sum1/1 -> Divide1/1
  Constant1/1 -> Divide1/2
  In1/1 -> Sum1/1, Delay1/1

== system flightController/Variant Subsystem/ANN/Subsystem/Subsystem13/Subsystem12 ==
  <Acel_z> : Inport
  Constant : Constant  Value=Normalization(24,2)
  Gain : Gain  Gain=1/(Normalization(24,1)-Normalization(24,2))
  Sum : Sum  Inputs=|+-
  Acceleracion Z : Outport
  wires:
  Sum/1 -> Gain/1
  <Acel_z>/1 -> Sum/1
  Constant/1 -> Sum/2
  Gain/1 -> Acceleracion Z/1

== system flightController/Variant Subsystem/ANN/Subsystem/Subsystem13/Subsystem13 ==
  In1 : Inport
  Constant1 : Constant  Value=Ts
  Delay1 : Delay  DelayLength=1  InitialCondition=0
  Divide1 : Product  Inputs=*/
  Sum1 : Sum  Inputs=|+-
  <Acel_Z> : Outport
  wires:
  Divide1/1 -> <Acel_Z>/1
  Delay1/1 -> Sum1/2
  Sum1/1 -> Divide1/1
  Constant1/1 -> Divide1/2
  In1/1 -> Sum1/1, Delay1/1

== system flightController/Variant Subsystem/ANN/Subsystem/Subsystem13/Subsystem14 ==
  <Acel_z> : Inport
  Constant : Constant  Value=Normalization(25,2)
  Gain : Gain  Gain=1/(Normalization(25,1)-Normalization(25,2))
  Sum : Sum  Inputs=|+-
  Acceleracion Z : Outport
  wires:
  Sum/1 -> Gain/1
  <Acel_z>/1 -> Sum/1
  Constant/1 -> Sum/2
  Gain/1 -> Acceleracion Z/1

== system flightController/Variant Subsystem/ANN/Subsystem/Subsystem13/Subsystem15 ==
  In1 : Inport
  Constant1 : Constant  Value=Ts
  Delay1 : Delay  DelayLength=1  InitialCondition=0
  Divide1 : Product  Inputs=*/
  Sum1 : Sum  Inputs=|+-
  <Acel_Z> : Outport
  wires:
  Divide1/1 -> <Acel_Z>/1
  Delay1/1 -> Sum1/2
  Sum1/1 -> Divide1/1
  Constant1/1 -> Divide1/2
  In1/1 -> Sum1/1, Delay1/1

== system flightController/Variant Subsystem/ANN/Subsystem/Subsystem13/Subsystem16 ==
  <Acel_z> : Inport
  Constant : Constant  Value=Normalization(26,2)
  Gain : Gain  Gain=1/(Normalization(26,1)-Normalization(26,2))
  Sum : Sum  Inputs=|+-
  Acceleracion Z : Outport
  wires:
  Sum/1 -> Gain/1
  <Acel_z>/1 -> Sum/1
  Constant/1 -> Sum/2
  Gain/1 -> Acceleracion Z/1

== system flightController/Variant Subsystem/ANN/Subsystem/Subsystem13/Subsystem2 ==
  <Z> : Inport
  Constant : Constant  Value=Normalization(2,2)
  Gain : Gain  Gain=1/(Normalization(2,1)-Normalization(2,2))
  Sum : Sum  Inputs=|+-
  Z : Outport
  wires:
  Constant/1 -> Sum/2
  Sum/1 -> Gain/1
  Gain/1 -> Z/1
  <Z>/1 -> Sum/1

== system flightController/Variant Subsystem/ANN/Subsystem/Subsystem13/Subsystem3 ==
  <Z> : Inport
  Constant : Constant  Value=Normalization(1,2)
  Gain : Gain  Gain=1/(Normalization(1,1)-Normalization(1,2))
  Sum : Sum  Inputs=|+-
  Z : Outport
  wires:
  Constant/1 -> Sum/2
  Sum/1 -> Gain/1
  Gain/1 -> Z/1
  <Z>/1 -> Sum/1

== system flightController/Variant Subsystem/ANN/Subsystem/Subsystem13/Subsystem4 ==
  <dz> : Inport
  Constant : Constant  Value=Normalization(4,2)
  Gain : Gain  Gain=1/(Normalization(4,1)-Normalization(4,2))
  Sum : Sum  Inputs=|+-
  Dz : Outport
  wires:
  Gain/1 -> Dz/1
  Constant/1 -> Sum/2
  <dz>/1 -> Sum/1
  Sum/1 -> Gain/1

== system flightController/Variant Subsystem/ANN/Subsystem/Subsystem13/Subsystem5 ==
  In1 : Inport
  Constant1 : Constant  Value=Ts
  Delay1 : Delay  DelayLength=1  InitialCondition=0
  Divide1 : Product  Inputs=*/
  Sum1 : Sum  Inputs=|+-
  <Acel_Z> : Outport
  wires:
  In1/1 -> Delay1/1, Sum1/1
  Constant1/1 -> Divide1/2
  Sum1/1 -> Divide1/1
  Delay1/1 -> Sum1/2
  Divide1/1 -> <Acel_Z>/1

== system flightController/Variant Subsystem/ANN/Subsystem/Subsystem13/Subsystem6 ==
  <Acel_z> : Inport
  Constant : Constant  Value=Normalization(18,2)
  Gain : Gain  Gain=1/(Normalization(18,1)-Normalization(18,2))
  Sum : Sum  Inputs=|+-
  Acceleracion Z : Outport
  wires:
  Gain/1 -> Acceleracion Z/1
  Constant/1 -> Sum/2
  <Acel_z>/1 -> Sum/1
  Sum/1 -> Gain/1

== system flightController/Variant Subsystem/ANN/Subsystem/Subsystem13/Subsystem7 ==
  <Z> : Inport
  Constant : Constant  Value=Normalization(3,2)
  Gain : Gain  Gain=1/(Normalization(3,1)-Normalization(3,2))
  Sum : Sum  Inputs=|+-
  Z : Outport
  wires:
  Constant/1 -> Sum/2
  Sum/1 -> Gain/1
  Gain/1 -> Z/1
  <Z>/1 -> Sum/1

== system flightController/Variant Subsystem/ANN/Subsystem/Subsystem13/Subsystem8 ==
  <dz> : Inport
  Constant : Constant  Value=Normalization(5,2)
  Gain : Gain  Gain=1/(Normalization(5,1)-Normalization(5,2))
  Sum : Sum  Inputs=|+-
  Dz : Outport
  wires:
  Sum/1 -> Gain/1
  <dz>/1 -> Sum/1
  Constant/1 -> Sum/2
  Gain/1 -> Dz/1

== system flightController/Variant Subsystem/ANN/Subsystem/Subsystem13/Subsystem9 ==
  <Z> : Inport
  Constant : Constant  Value=Normalization(6,2)
  Gain : Gain  Gain=1/(Normalization(6,1)-Normalization(6,2))
  Sum : Sum  Inputs=|+-
  Z : Outport
  wires:
  Constant/1 -> Sum/2
  Sum/1 -> Gain/1
  Gain/1 -> Z/1
  <Z>/1 -> Sum/1

== system flightController/Variant Subsystem/ANN/Subsystem/Subsystem3/Subsystem ==
  <Z_r> : Inport
  Constant : Constant  Value=Normalization(8,2)
  Gain : Gain  Gain=1/(Normalization(8,1)-Normalization(8,2))
  Sum : Sum  Inputs=|+-
  Z_r : Outport
  wires:
  <Z_r>/1 -> Sum/1
  Sum/1 -> Gain/1
  Constant/1 -> Sum/2
  Gain/1 -> Z_r/1

== system flightController/Variant Subsystem/ANN/Subsystem/Subsystem3/Subsystem1 ==
  In1 : Inport
  Constant1 : Constant  Value=Ts
  Delay1 : Delay  DelayLength=1  InitialCondition=0
  Divide1 : Product  Inputs=*/
  Sum1 : Sum  Inputs=|+-
  Out1 : Outport
  wires:
  In1/1 -> Delay1/1, Sum1/1
  Constant1/1 -> Divide1/2
  Sum1/1 -> Divide1/1
  Delay1/1 -> Sum1/2
  Divide1/1 -> Out1/1

== system flightController/Variant Subsystem/ANN/Subsystem/Subsystem3/Subsystem2 ==
  <Dz_r> : Inport
  Constant : Constant  Value=Normalization(11,2)
  Gain : Gain  Gain=1/(Normalization(11,1)-Normalization(11,2))
  Sum : Sum  Inputs=|+-
  Dz_r : Outport
  wires:
  <Dz_r>/1 -> Sum/1
  Sum/1 -> Gain/1
  Constant/1 -> Sum/2
  Gain/1 -> Dz_r/1

== system flightController/Variant Subsystem/ANN/Subsystem/Subsystem3/Subsystem3 ==
  <Z_r> : Inport
  Constant : Constant  Value=0
  Constant1 : Constant  Commented=on  Value=Normalization(5,2)
  Gain : Gain  Commented=on  Gain=1/(Normalization(10,1)-Normalization(10,2))
  Gain1 : Gain
  Sum : Sum  Inputs=|+-
  Z_r : Outport
  wires:
  <Z_r>/1 -> Sum/1
  Constant/1 -> Sum/2
  Sum/1 -> Gain1/1
  Gain1/1 -> Z_r/1

== system flightController/Variant Subsystem/ANN/Subsystem/Subsystem3/Subsystem4 ==
  <Z_r> : Inport
  Constant : Constant  Value=Normalization(10,2)
  Gain : Gain  Commented=on  Gain=1/(Normalization(11,1)-Normalization(11,2))
  Gain1 : Gain  Gain=0
  Sum : Sum  Inputs=|+-
  Z_r : Outport
  wires:
  <Z_r>/1 -> Sum/1
  Constant/1 -> Sum/2
  Sum/1 -> Gain1/1
  Gain1/1 -> Z_r/1

== system flightController/Variant Subsystem/ANN/Subsystem/Subsystem3/Subsystem5 ==
  <Z_r> : Inport
  Constant : Constant  Value=Normalization(9,2)
  Gain : Gain  Commented=on  Gain=1/(Normalization(7,1)-Normalization(7,2))
  Gain1 : Gain  Gain=0
  Sum : Sum  Inputs=|+-
  Z_r : Outport
  wires:
  <Z_r>/1 -> Sum/1
  Constant/1 -> Sum/2
  Sum/1 -> Gain1/1
  Gain1/1 -> Z_r/1

== system flightController/Variant Subsystem/ANN/Subsystem/Subsystem3/Subsystem6 ==
  <Dz_r> : Inport
  Constant : Constant  Value=Normalization(14,2)
  Gain : Gain  Commented=on  Gain=1/(Normalization(14,1)-Normalization(14,2))
  Gain1 : Gain
  Sum : Sum  Inputs=|+-
  Dz_r : Outport
  wires:
  <Dz_r>/1 -> Sum/1
  Constant/1 -> Sum/2
  Sum/1 -> Gain1/1
  Gain1/1 -> Dz_r/1

== system flightController/Variant Subsystem/ANN/Subsystem/Subsystem3/Subsystem7 ==
  <Dz_r> : Inport
  Constant : Constant  Value=Normalization(15,2)
  Gain : Gain  Gain=1/(Normalization(15,1)-Normalization(15,2))
  Sum : Sum  Inputs=|+-
  Dz_r : Outport
  wires:
  <Dz_r>/1 -> Sum/1
  Sum/1 -> Gain/1
  Constant/1 -> Sum/2
  Gain/1 -> Dz_r/1

== system flightController/Variant Subsystem/ANN/Subsystem/Subsystem3/Subsystem8 ==
  <Dz_r> : Inport
  Constant : Constant  Value=Normalization(16,2)
  Gain : Gain  Gain=1/(Normalization(16,1)-Normalization(16,2))
  Sum : Sum  Inputs=|+-
  Dz_r : Outport
  wires:
  <Dz_r>/1 -> Sum/1
  Sum/1 -> Gain/1
  Constant/1 -> Sum/2
  Gain/1 -> Dz_r/1

== system flightController/Variant Subsystem/ANN_Feedback/Subsystem1/Subsystem/Subsystem1 ==
  <Pressure Altitud> : Inport
  Constant : Constant  Value=Normalization(13,2)
  Gain : Gain  Gain=1/(Normalization(13,1)-Normalization(13,2))
  Sum : Sum  Inputs=|+-
  Pressure Altitud : Outport
  wires:
  <Pressure Altitud>/1 -> Sum/1
  Sum/1 -> Gain/1
  Constant/1 -> Sum/2
  Gain/1 -> Pressure Altitud/1

== system flightController/Variant Subsystem/ANN_Feedback/Subsystem1/Subsystem/Subsystem2 ==
  <Pressure Altitud> : Inport
  Constant : Constant  Value=Normalization(23,2)
  Gain : Gain  Gain=1/(Normalization(23,1)-Normalization(23,2))
  Sum : Sum  Inputs=|+-
  Pressure Altitud : Outport
  wires:
  <Pressure Altitud>/1 -> Sum/1
  Sum/1 -> Gain/1
  Constant/1 -> Sum/2
  Gain/1 -> Pressure Altitud/1

== system flightController/Variant Subsystem/ANN_Feedback/Subsystem1/Subsystem/Subsystem3 ==
  <Pressure Altitud> : Inport
  Constant : Constant  Value=Normalization(17,2)
  Gain : Gain  Gain=1/(Normalization(17,1)-Normalization(17,2))
  Sum : Sum  Inputs=|+-
  Pressure Altitud : Outport
  wires:
  <Pressure Altitud>/1 -> Sum/1
  Sum/1 -> Gain/1
  Constant/1 -> Sum/2
  Gain/1 -> Pressure Altitud/1

== system flightController/Variant Subsystem/ANN_Feedback/Subsystem1/Subsystem/Subsystem4 ==
  <Ac_Dz> : Inport
  Constant : Constant  Value=Normalization(21,2)
  Gain : Gain  Gain=1/(Normalization(21,1)-Normalization(21,2))
  Sum : Sum  Inputs=|+-
  Ac_Dz : Outport
  wires:
  Gain/1 -> Ac_Dz/1
  Constant/1 -> Sum/2
  Sum/1 -> Gain/1
  <Ac_Dz>/1 -> Sum/1

== system flightController/Variant Subsystem/ANN_Feedback/Subsystem1/Subsystem/Subsystem5 ==
  <Ac_Dz> : Inport
  Constant : Constant  Value=Normalization(20,2)
  Gain : Gain  Gain=1/(Normalization(20,1)-Normalization(20,2))
  Sum : Sum  Inputs=|+-
  Ac_Dz : Outport
  wires:
  <Ac_Dz>/1 -> Sum/1
  Sum/1 -> Gain/1
  Constant/1 -> Sum/2
  Gain/1 -> Ac_Dz/1

== system flightController/Variant Subsystem/ANN_Feedback/Subsystem1/Subsystem/Subsystem7 ==
  <Ac_Dz> : Inport
  Constant : Constant  Value=Normalization(22,2)
  Gain : Gain  Gain=1/(Normalization(22,1)-Normalization(22,2))
  Sum : Sum  Inputs=|+-
  Ac_Dz : Outport
  wires:
  <Ac_Dz>/1 -> Sum/1
  Sum/1 -> Gain/1
  Constant/1 -> Sum/2
  Gain/1 -> Ac_Dz/1

== system flightController/Variant Subsystem/ANN_Feedback/Subsystem1/Subsystem/Subsystem8 ==
  <Pressure Altitud> : Inport
  Constant : Constant  Value=Normalization(14,2)
  Gain : Gain  Gain=1/(Normalization(14,1)-Normalization(14,2))
  Sum : Sum  Inputs=|+-
  Pressure Altitud : Outport
  wires:
  <Pressure Altitud>/1 -> Sum/1
  Sum/1 -> Gain/1
  Constant/1 -> Sum/2
  Gain/1 -> Pressure Altitud/1

== system flightController/Variant Subsystem/ANN_Feedback/Subsystem1/Subsystem/Subsystem9 ==
  <Sonar Altitud> : Inport
  Constant : Constant  Value=Normalization(16,2)
  Gain : Gain  Gain=1/(Normalization(16,1)-Normalization(16,2))
  Scope : Scope
  Sum : Sum  Inputs=|+-
  Sonar Altitud : Outport
  wires:
  <Sonar Altitud>/1 -> Scope/1, Sum/1
  Sum/1 -> Gain/1
  Constant/1 -> Sum/2
  Gain/1 -> Sonar Altitud/1

== system flightController/Variant Subsystem/ANN_Feedback/Subsystem1/Subsystem10/Subsystem ==
  <Z_r> : Inport
  Constant : Constant  Value=Normalization(10,2)
  Gain : Gain  Gain=1/(Normalization(10,1)-Normalization(10,2))
  Sum : Sum  Inputs=|+-
  Z_r : Outport
  wires:
  <Z_r>/1 -> Sum/1
  Sum/1 -> Gain/1
  Constant/1 -> Sum/2
  Gain/1 -> Z_r/1

== system flightController/Variant Subsystem/ANN_Feedback/Subsystem1/Subsystem10/Subsystem2 ==
  <Dz_r> : Inport
  Constant : Constant  Value=Normalization(14,2)
  Gain : Gain  Gain=1/(Normalization(14,1)-Normalization(14,2))
  Sum : Sum  Inputs=|+-
  Dz_r : Outport
  wires:
  <Dz_r>/1 -> Sum/1
  Sum/1 -> Gain/1
  Constant/1 -> Sum/2
  Gain/1 -> Dz_r/1

== system flightController/Variant Subsystem/ANN_Feedback/Subsystem1/Subsystem10/Subsystem3 ==
  <Z> : Inport
  Constant : Constant  Value=Normalization(2,2)
  Gain : Gain  Gain=1/(Normalization(2,1)-Normalization(2,2))
  Sum : Sum  Inputs=|+-
  Z : Outport
  wires:
  Constant/1 -> Sum/2
  Sum/1 -> Gain/1
  Gain/1 -> Z/1
  <Z>/1 -> Sum/1

== system flightController/Variant Subsystem/ANN_Feedback/Subsystem1/Subsystem10/Subsystem4 ==
  <dz> : Inport
  Constant : Constant  Value=Normalization(5,2)
  Gain : Gain  Gain=1/(Normalization(5,1)-Normalization(5,2))
  Sum : Sum  Inputs=|+-
  Dz : Outport
  wires:
  Gain/1 -> Dz/1
  Constant/1 -> Sum/2
  <dz>/1 -> Sum/1
  Sum/1 -> Gain/1

== system flightController/Variant Subsystem/ANN_Feedback/Subsystem1/Subsystem10/Subsystem6 ==
  <Acel_z> : Inport
  Constant : Constant  Value=Normalization(30,2)
  Gain : Gain  Gain=1/(Normalization(30,1)-Normalization(30,2))
  Sum : Sum  Inputs=|+-
  Acceleracion Z : Outport
  wires:
  Gain/1 -> Acceleracion Z/1
  Constant/1 -> Sum/2
  <Acel_z>/1 -> Sum/1
  Sum/1 -> Gain/1

== system flightController/Variant Subsystem/ANN_Feedback/Subsystem1/Subsystem10/Subsystem7 ==
  <Ac_Dz> : Inport
  Constant : Constant  Value=Normalization(18,2)
  Gain : Gain  Gain=1/(Normalization(18,1)-Normalization(18,2))
  Sum : Sum  Inputs=|+-
  Ac_Dz : Outport
  wires:
  <Ac_Dz>/1 -> Sum/1
  Sum/1 -> Gain/1
  Constant/1 -> Sum/2
  Gain/1 -> Ac_Dz/1

== system flightController/Variant Subsystem/ANN_Feedback/Subsystem1/Subsystem10/Subsystem8 ==
  <Pressure Altitud> : Inport
  Constant : Constant  Value=Normalization(26,2)
  Gain : Gain  Gain=1/(Normalization(26,1)-Normalization(26,2))
  Sum : Sum  Inputs=|+-
  Pressure Altitud : Outport
  wires:
  <Pressure Altitud>/1 -> Sum/1
  Sum/1 -> Gain/1
  Constant/1 -> Sum/2
  Gain/1 -> Pressure Altitud/1

== system flightController/Variant Subsystem/ANN_Feedback/Subsystem1/Subsystem10/Subsystem9 ==
  <Sonar Altitud> : Inport
  Constant : Constant  Value=Normalization(22,2)
  Gain : Gain  Gain=1/(Normalization(22,1)-Normalization(22,2))
  Sum : Sum  Inputs=|+-
  Sonar Altitud : Outport
  wires:
  <Sonar Altitud>/1 -> Sum/1
  Sum/1 -> Gain/1
  Constant/1 -> Sum/2
  Gain/1 -> Sonar Altitud/1

== system flightController/Variant Subsystem/ANN_Feedback/Subsystem1/Subsystem11/Subsystem ==
  <Z_r> : Inport
  Constant : Constant  Value=Normalization(10,2)
  Gain : Gain  Gain=1/(Normalization(10,1)-Normalization(10,2))
  Sum : Sum  Inputs=|+-
  Z_r : Outport
  wires:
  <Z_r>/1 -> Sum/1
  Sum/1 -> Gain/1
  Constant/1 -> Sum/2
  Gain/1 -> Z_r/1

== system flightController/Variant Subsystem/ANN_Feedback/Subsystem1/Subsystem11/Subsystem2 ==
  <Dz_r> : Inport
  Constant : Constant  Value=Normalization(14,2)
  Gain : Gain  Gain=1/(Normalization(14,1)-Normalization(14,2))
  Sum : Sum  Inputs=|+-
  Dz_r : Outport
  wires:
  <Dz_r>/1 -> Sum/1
  Sum/1 -> Gain/1
  Constant/1 -> Sum/2
  Gain/1 -> Dz_r/1

== system flightController/Variant Subsystem/ANN_Feedback/Subsystem1/Subsystem11/Subsystem3 ==
  <Z> : Inport
  Constant : Constant  Value=Normalization(3,2)
  Gain : Gain  Gain=1/(Normalization(3,1)-Normalization(3,2))
  Sum : Sum  Inputs=|+-
  Z : Outport
  wires:
  Constant/1 -> Sum/2
  Sum/1 -> Gain/1
  Gain/1 -> Z/1
  <Z>/1 -> Sum/1

== system flightController/Variant Subsystem/ANN_Feedback/Subsystem1/Subsystem11/Subsystem4 ==
  <dz> : Inport
  Constant : Constant  Value=Normalization(6,2)
  Gain : Gain  Gain=1/(Normalization(6,1)-Normalization(6,2))
  Sum : Sum  Inputs=|+-
  Dz : Outport
  wires:
  Gain/1 -> Dz/1
  Constant/1 -> Sum/2
  <dz>/1 -> Sum/1
  Sum/1 -> Gain/1

== system flightController/Variant Subsystem/ANN_Feedback/Subsystem1/Subsystem11/Subsystem6 ==
  <Acel_z> : Inport
  Constant : Constant  Value=Normalization(30,2)
  Gain : Gain  Gain=1/(Normalization(30,1)-Normalization(30,2))
  Sum : Sum  Inputs=|+-
  Acceleracion Z : Outport
  wires:
  Gain/1 -> Acceleracion Z/1
  Constant/1 -> Sum/2
  <Acel_z>/1 -> Sum/1
  Sum/1 -> Gain/1

== system flightController/Variant Subsystem/ANN_Feedback/Subsystem1/Subsystem11/Subsystem7 ==
  <Ac_Dz> : Inport
  Constant : Constant  Value=Normalization(18,2)
  Gain : Gain  Gain=1/(Normalization(18,1)-Normalization(18,2))
  Sum : Sum  Inputs=|+-
  Ac_Dz : Outport
  wires:
  <Ac_Dz>/1 -> Sum/1
  Sum/1 -> Gain/1
  Constant/1 -> Sum/2
  Gain/1 -> Ac_Dz/1

== system flightController/Variant Subsystem/ANN_Feedback/Subsystem1/Subsystem11/Subsystem8 ==
  <Pressure Altitud> : Inport
  Constant : Constant  Value=Normalization(26,2)
  Gain : Gain  Gain=1/(Normalization(26,1)-Normalization(26,2))
  Sum : Sum  Inputs=|+-
  Pressure Altitud : Outport
  wires:
  <Pressure Altitud>/1 -> Sum/1
  Sum/1 -> Gain/1
  Constant/1 -> Sum/2
  Gain/1 -> Pressure Altitud/1

== system flightController/Variant Subsystem/ANN_Feedback/Subsystem1/Subsystem11/Subsystem9 ==
  <Sonar Altitud> : Inport
  Constant : Constant  Value=Normalization(22,2)
  Gain : Gain  Gain=1/(Normalization(22,1)-Normalization(22,2))
  Sum : Sum  Inputs=|+-
  Sonar Altitud : Outport
  wires:
  <Sonar Altitud>/1 -> Sum/1
  Sum/1 -> Gain/1
  Constant/1 -> Sum/2
  Gain/1 -> Sonar Altitud/1

== system flightController/Variant Subsystem/ANN_Feedback/Subsystem1/Subsystem12/Subsystem ==
  <Z_r> : Inport
  Constant : Constant  Value=Normalization(10,2)
  Gain : Gain  Gain=1/(Normalization(10,1)-Normalization(10,2))
  Sum : Sum  Inputs=|+-
  Z_r : Outport
  wires:
  Gain/1 -> Z_r/1
  Constant/1 -> Sum/2
  Sum/1 -> Gain/1
  <Z_r>/1 -> Sum/1

== system flightController/Variant Subsystem/ANN_Feedback/Subsystem1/Subsystem12/Subsystem2 ==
  <Dz_r> : Inport
  Constant : Constant  Value=Normalization(14,2)
  Gain : Gain  Gain=1/(Normalization(14,1)-Normalization(14,2))
  Sum : Sum  Inputs=|+-
  Dz_r : Outport
  wires:
  Gain/1 -> Dz_r/1
  Constant/1 -> Sum/2
  Sum/1 -> Gain/1
  <Dz_r>/1 -> Sum/1
